simulink model "Problem3"  (R2020b)
settings: Solver=ode45  StartTime=0.0  StopTime=10.0  RelTol=1e-3
PostLoadFcn:
  | Kp=17.9947607768602;
  | Ki=41.8923134387203;
  | Kd=-0.685067684451754;
  | N=3.3394404818866;
model workspace (MAT data in the model file):
  J = Simulink.Parameter
  J.Value = 0.01
  J.DataType = 'auto'
  J.Dimensions = [1 1]
  K = Simulink.Parameter
  K.Value = 0.0274
  K.DataType = 'auto'
  K.Dimensions = [1 1]
  Kd = Simulink.Parameter
  Kd.Value = -0.685067684452
  Kd.DataType = 'auto'
  Kd.Dimensions = [1 1]
  Ki = Simulink.Parameter
  Ki.Value = 41.8923134387
  Ki.DataType = 'auto'
  Ki.Dimensions = [1 1]
  Kp = Simulink.Parameter
  Kp.Value = 17.9947607769
  Kp.DataType = 'auto'
  Kp.Dimensions = [1 1]
  L = Simulink.Parameter
  L.Value = 0.5
  L.DataType = 'auto'
  L.Dimensions = [1 1]
  N = Simulink.Parameter
  N.Value = 3.33944048189
  N.DataType = 'auto'
  N.Dimensions = [1 1]
  R = Simulink.Parameter
  R.Value = 1
  R.DataType = 'auto'
  R.Dimensions = [1 1]
  b = Simulink.Parameter
  b.Value = 0.1
  b.DataType = 'auto'
  b.Dimensions = [1 1]
undefined symbols (not defined in the file): sigbuilder_block
settings Model: OrderedModelArguments=off  Creator=Hp  LastModifiedBy=Hp

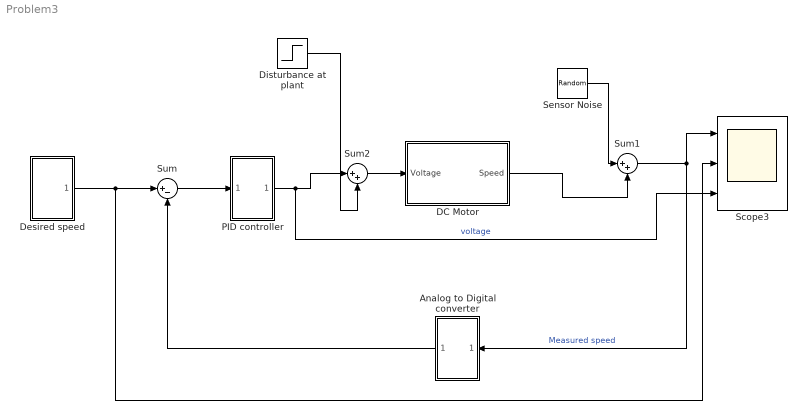
== system Problem3 ==
  Analog to Digital converter : Subsystem
  DC Motor : Subsystem
  Desired speed : Subsystem
  Disturbance at plant : Step  SampleTime=0
  PID controller : Subsystem
  Scope3 : Scope  NumInputPorts=3
  Sensor Noise : RandomNumber  SampleTime=0.1
  Sum : Sum  Inputs=|+-
  Sum1 : Sum  Inputs=|++
  Sum2 : Sum  Inputs=|++
  wires:
  Desired speed/1(Speed) -> Scope3/2, Sum/1
  Sum1/1 -> Analog to Digital converter/1(Inport), Scope3/1  "Measured speed"
  Analog to Digital converter/1(Outport) -> Sum/2
  Sensor Noise/1 -> Sum1/1
  Sum/1 -> PID controller/1(Inport)
  Disturbance at plant/1 -> Sum2/2
  PID controller/1(Outport) -> Scope3/3, Sum2/1  "voltage"
  DC Motor/1(Speed) -> Sum1/2
  Sum2/1 -> DC Motor/1(Voltage)

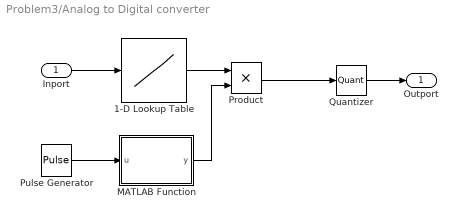
== system Problem3/Analog to Digital converter ==
  Inport : Inport
  1-D Lookup Table : Lookup_n-D  NumberOfTableDimensions=1  BreakpointsForDimension1=[5 6 7]  Table=[2 3 4]  InternalRulePriority=Speed  RndMeth=Simplest  InputSameDT=on
  MATLAB Function : MATLAB Function  TreatAsAtomicUnit=on
  Product : Product
  Pulse Generator : DiscretePulseGenerator  PulseType=Time based  Amplitude=10  Period=0.2  PulseWidth=2  PhaseDelay=0.5
  Quantizer : Quantizer  QuantizationInterval=1
  Outport : Outport
  wires:
  Product/1 -> Quantizer/1
  Quantizer/1 -> Outport/1
  Inport/1 -> 1-D Lookup Table/1
  1-D Lookup Table/1 -> Product/1
  MATLAB Function/1(y) -> Product/2
  Pulse Generator/1 -> MATLAB Function/1(u)

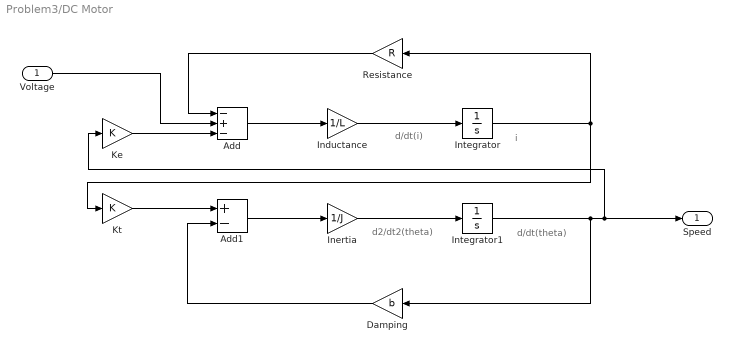
== system Problem3/DC Motor ==
  note: i
  note: d/dt(theta)
  note: d/dt(i)
  note: d2/dt2(theta)
  Voltage : Inport
  Add : Sum  Inputs=-+-
  Add1 : Sum  Inputs=+-
  Damping : Gain  Gain=b
  Inductance : Gain  Gain=1/L
  Inertia : Gain  Gain=1/J
  Integrator : Integrator
  Integrator1 : Integrator
  Ke : Gain  Gain=K
  Kt : Gain  Gain=K
  Resistance : Gain  Gain=R
  Speed : Outport
  wires:
  Damping/1 -> Add1/2
  Resistance/1 -> Add/1
  Add/1 -> Inductance/1
  Kt/1 -> Add1/1
  Integrator/1 -> Resistance/1, Kt/1
  Integrator1/1 -> Damping/1, Speed/1, Ke/1
  Inductance/1 -> Integrator/1
  Add1/1 -> Inertia/1
  Voltage/1 -> Add/2
  Ke/1 -> Add/3
  Inertia/1 -> Integrator1/1

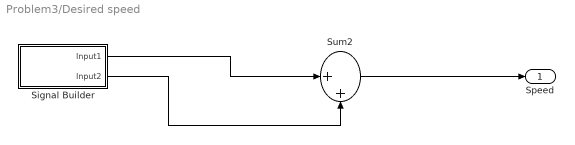
== system Problem3/Desired speed ==
  Signal Builder : Subsystem  Tag=STV Subsys  LoadFcn=sigbuilder_block('load');  StartFcn=sigbuilder_block('start');  StopFcn=sigbuilder_block('stop');  ClipboardFcn=sigbuilder_block('clipboard');  mask(Sigbuilder block){tuvar=[0:10]}
      mask help: Simulink:masks:SigbuilderBlock_MD
      mask init:
      | if ~strcmp(get_param(bdroot(gcbh),'SimulationStatus'),'stopped') tuvar = sigbuilder_block('maskInit'); end
      settings: CopyFcn=sigbuilder_block('copy');  DeleteFcn=sigbuilder_block('delete');  ModelCloseFcn=sigbuilder_block('modelClose');  PreSaveFcn=sigbuilder_block('preSave');  PauseFcn=sigbuilder_block('pause');  ContinueFcn=sigbuilder_block('continue');  NameChangeFcn=sigbuilder_block('namechange');  OpenFcn=sigbuilder_block('open',[404 117.5 550.5 362.5 ]);  CloseFcn=sigbuilder_block('close');
      mask Display: plot(0, 0, 100, 100,[2, 2, 32, 32, 2], [68, 8, 8, 68, 68],[32, 2], [38, 38], [32, 19, 2],[53, 60, 44], [32, 17, 17, 2],[16, 16, 31, 31]);txt = getActiveGroup(gcbh);text(2, 100, txt,'verticalAlignment', 'top');
  Sum2 : Sum  Inputs=|++
  Speed : Outport
  wires:
  Signal Builder/1(Input1) -> Sum2/1
  Sum2/1 -> Speed/1
  Signal Builder/2(Input2) -> Sum2/2

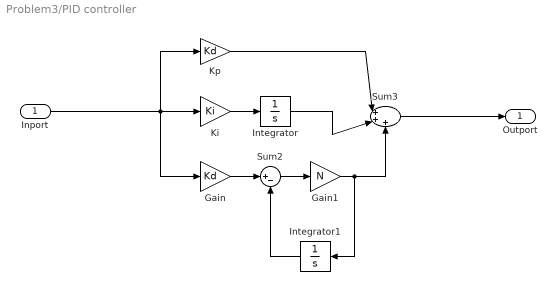
== system Problem3/PID controller ==
  Inport : Inport
  Gain : Gain  Gain=Kd
  Gain1 : Gain  Gain=N
  Integrator : Integrator
  Integrator1 : Integrator
  Ki : Gain  Gain=Ki
  Kp : Gain  Gain=Kd
  Sum2 : Sum  Inputs=|+-
  Sum3 : Sum  Inputs=|+++
  Outport : Outport
  wires:
  Integrator1/1 -> Sum2/2
  Gain/1 -> Sum2/1
  Inport/1 -> Gain/1, Kp/1, Ki/1
  Gain1/1 -> Integrator1/1, Sum3/3
  Sum2/1 -> Gain1/1
  Sum3/1 -> Outport/1
  Integrator/1 -> Sum3/2
  Ki/1 -> Integrator/1
  Kp/1 -> Sum3/1

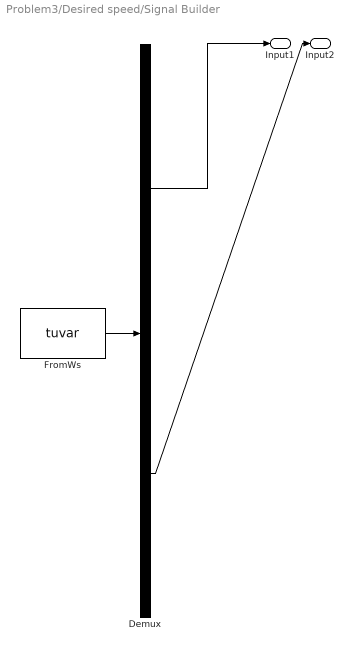
== system Problem3/Desired speed/Signal Builder ==
  Demux : Demux  Tag=STV Demux  Outputs=2
      settings: DisplayOption=none
  FromWs : FromWorkspace  Tag=STV FromWs  VariableName=tuvar
      SigBuilderData=|
      | common.afterFinalStr = 'Extrapolate'
      | common.sampleTime = 0
      | dataSet.timeRange = [0 10]
      | dataSet.name = 'Group 1'
      | sbobj.Groups.Name = 'Group 1'
      | sbobj.Groups.Signals(1).Name = 'Input1'
      | sbobj.Groups.Signals(1).XData = [0 5 5 10]
      | sbobj.Groups.Signals(1).YData = [0 0 1 1]
      | sbobj.Groups.Signals(2).Name = 'Input2'
      | sbobj.Groups.Signals(2).XData = [0 5 5 10]
      | sbobj.Groups.Signals(2).YData = [0 0 -0.058 -0.0585]
  Input1 : Outport  Tag=STV Outport
  Input2 : Outport  Tag=STV Outport  Port=2
  wires:
  FromWs/1 -> Demux/1
  Demux/1 -> Input1/1
  Demux/2 -> Input2/1

== matlab function Problem3/Analog to Digital converter/MATLAB Function ==
  data: u input; y output
function y = fcn(u)
if(u>1)
    y=1;
else
    y=0;
end
end
